simulink model "Exp32"  (R2025b)
settings: Solver=VariableStepAuto  StartTime=0.0  StopTime=1  RelTol=1e-3
libraries: commrandsrc3 x2, dspsigops x2, commdigbbndcpm2 x1, commrflib2 x1, commdigbbndpm3 x1
settings Model: Creator=pc  LastModifiedBy=pc

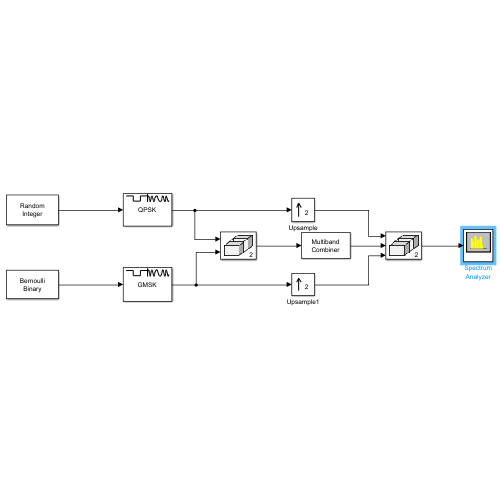
[thumbnail: Simulink's stored preview of the top-level diagram]
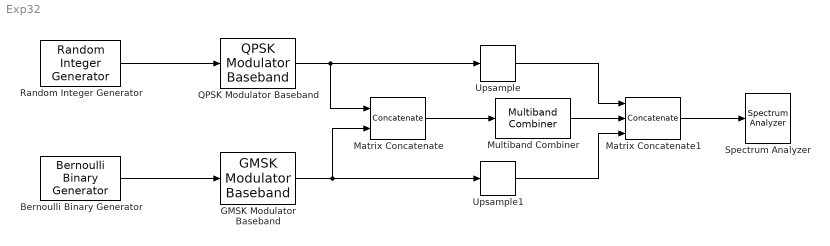
== system Exp32 ==
  Bernoulli Binary Generator : commrandsrc3/Bernoulli Binary Generator  ProbabilityOfZero=0.5  SeedSource=Auto  Seed=0  SampleTime=2e-5  SamplesPerFrame=1  OutputDataType=double  SimulateUsing=Interpreted execution
  GMSK Modulator Baseband : commdigbbndcpm2/GMSK Modulator Baseband  inputType=Bit  BT=.3  pulseLength=4  preHistory=1  phaseOffset=0  samplesPerSymbol=2  RateOptions=Enforce single-rate processing  outDataType=double
  Matrix Concatenate : Concatenate  Mode=Multidimensional array  ConcatenateDimension=2
  Matrix Concatenate1 : Concatenate  NumInputs=3  Mode=Multidimensional array  ConcatenateDimension=2
  Multiband Combiner : commrflib2/Multiband Combiner  InputSampleRate=100e3  FrequencyOffsets=[-50e3, 50e3]  RateOption=Enforce single-rate processing  OutputSampleRateOption=Specify via property  OutputSampleRate=200e3
  QPSK Modulator Baseband : commdigbbndpm3/QPSK Modulator Baseband  InType=Integer  Enc=Gray  Ph=pi/4  outDtype=double  outWordLen=16  outUDDataType=sfix(16)  outFracLenMode=Best precision  outFracLen=15  outDataTypeStr=double  outLastDataTypeStr=double
  Random Integer Generator : commrandsrc3/Random Integer Generator  SetSize=4  SeedSource=Auto  Seed=0  SampleTime=2e-5  SamplesPerFrame=2  OutputDataType=double  SimulateUsing=Interpreted execution
  Spectrum Analyzer : SpectrumAnalyzer  WindowPosition=[1.000000,49.000000,1366.000000,697.000000,]  ScopeFrameLocation=window  SampleRate=44.1e3  FrequencyScale=Log  WindowInvariantSamplesPerUpdate=on  FrequencySpan=Start and stop frequencies  StartFrequency=20  StopFrequency=20e3  YLimits=[-28.6777 0.0783]  SelectedToolstripTab=spectrumAnalyzerToolstrip.spectrumTab
  Upsample : dspsigops/Upsample  FactorSource=Dialog parameter  N=2  Nmax=16  phase=0  InputProcessing=Columns as channels (frame based)  RateOptions=Enforce single-rate processing  ic=0  mode=Unused parameter value
      settings: LibrarySourceBlock=dsphdlsupportsigops/Upsample
  Upsample1 : dspsigops/Upsample  FactorSource=Dialog parameter  N=2  Nmax=16  phase=0  InputProcessing=Columns as channels (frame based)  RateOptions=Enforce single-rate processing  ic=0  mode=Unused parameter value
      settings: LibrarySourceBlock=dsphdlsupportsigops/Upsample
  wires:
  Random Integer Generator/1 -> QPSK Modulator Baseband/1
  QPSK Modulator Baseband/1 -> Matrix Concatenate/1, Upsample/1
  GMSK Modulator Baseband/1 -> Matrix Concatenate/2, Upsample1/1
  Matrix Concatenate/1 -> Multiband Combiner/1
  Upsample/1 -> Matrix Concatenate1/1
  Upsample1/1 -> Matrix Concatenate1/3
  Multiband Combiner/1 -> Matrix Concatenate1/2
  Matrix Concatenate1/1 -> Spectrum Analyzer/1
  Bernoulli Binary Generator/1 -> GMSK Modulator Baseband/1
